simulink library "Valve_fn"  (Simulink 8.2)
settings: Solver=ode45  StartTime=0.0  StopTime=10.0  RelTol=1e-3
undefined symbols (not defined in the file): DPConstant, DPLinear, DPQuadratic, ID, Pressure
libraries: carnot x1
settings Model: Creator=lena.frank  LastModifiedBy=drhf

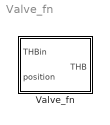
== system Valve_fn ==
  Valve_fn : Subsystem  mask(valve with Kv function){kv=0.7, kvs=0.9, op=0.5}
      mask prompts: kv "Kv value"; kvs "Kvs value"; op "Operation point [0..1]"
      mask help:
      | The block calculates the pressure drop at a valve. The characteristic is defined the function:
      | QUA = 2.8e6*(kv/(kvs*(2/(1+exp(-2/op*u(1)))-1)))^2
      | dp = QUA * mdot^2
      mask Help: web(fullfile(path_carnot('help'),'Valve_fn.html'),'-helpbrowser')
      mask Display: plot(-15,0,115,100,[30,70,70,30,30],[60,40,60,40,60],[60,40],[80,80],[50,50],[50,80])

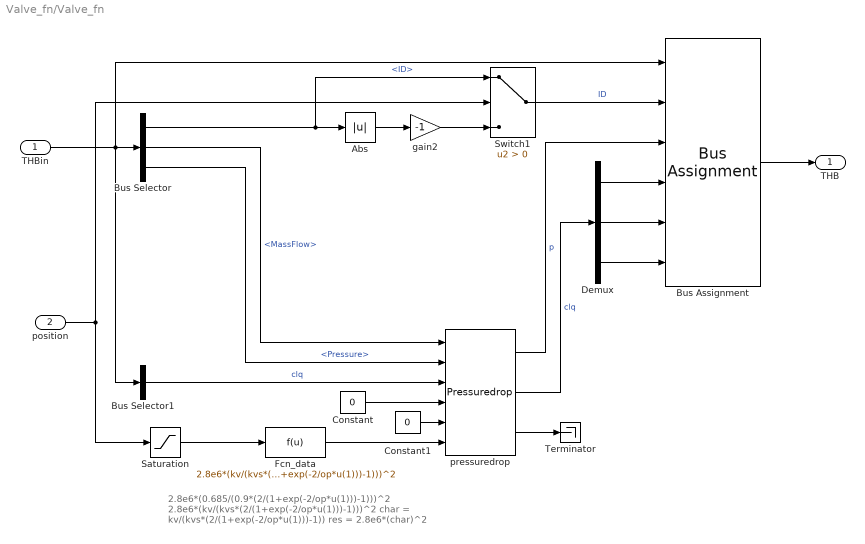
== system Valve_fn/Valve_fn ==
  note: 2.8e6*(0.685/(0.9*(2/(1+exp(-2/op*u(1)))-1)))^2
      | 2.8e6*(kv/(kvs*(2/(1+exp(-2/op*u(1)))-1)))^2
      |
      | char = kv/(kvs*(2/(1+exp(-2/op*u(1)))-1))
      | res = 2.8e6*(char)^2
  THBin : Inport
  position : Inport  Port=2
  Abs : Abs
  Bus Assignment : BusAssignment  AssignedSignals=ID,Pressure,DPConstant,DPLinear,DPQuadratic
  Bus Selector : BusSelector  OutputSignals=ID,MassFlow,Pressure
  Bus Selector1 : BusSelector  OutputSignals=DPConstant,DPLinear,DPQuadratic  OutputAsBus=on
  Constant : Constant  Value=0
  Constant1 : Constant  Value=0
  Demux : Demux  Outputs=3
  Fcn_data : Fcn  Expr=2.8e6*(kv/(kvs*(2/(1+exp(-2/op*u(1)))-1)))^2
  Saturation : Saturate  UpperLimit=1  LowerLimit=1e-9
  Switch1 : Switch  Criteria=u2 > Threshold  SaturateOnIntegerOverflow=on  InputSameDT=on
  Terminator : Terminator
  gain2 : Gain  Gain=-1  SaturateOnIntegerOverflow=on  OutDataTypeStr=Inherit: Same as input  ParamDataTypeStr=Inherit: Same as input
  pressuredrop : carnot/Basic/Pressure_Drop/Pressuredrop
  THB : Outport  InitialOutput=0
  wires:
  Saturation/1 -> Fcn_data/1
  Fcn_data/1 -> pressuredrop/6
  Demux/3 -> Bus Assignment/6
  Demux/2 -> Bus Assignment/5
  Demux/1 -> Bus Assignment/4
  Bus Assignment/1 -> THB/1
  THBin/1 -> Bus Assignment/1, Bus Selector1/1, Bus Selector/1
  pressuredrop/3 -> Terminator/1
  Constant1/1 -> pressuredrop/5
  Constant/1 -> pressuredrop/4
  pressuredrop/2 -> Demux/1  "clq"
  Bus Selector/3 -> pressuredrop/2  "<Pressure>"
  Abs/1 -> gain2/1
  Switch1/1 -> Bus Assignment/2  "ID"
  Bus Selector/2 -> pressuredrop/1  "<MassFlow>"
  pressuredrop/1 -> Bus Assignment/3  "p"
  Bus Selector1/1 -> pressuredrop/3  "clq"
  position/1 -> Switch1/2, Saturation/1
  Bus Selector/1 -> Abs/1, Switch1/1  "<ID>"
  gain2/1 -> Switch1/3
